simulink model "Energy_consumption_model_V3"  (R2022b)
settings: Solver=VariableStepAuto  StartTime=0.0  StopTime=110  RelTol=1e-3
undefined symbols (not defined in the file or in its folder): arr_db, arr_fg, arr_l, arr_lm, arr_mc1, arr_mc2, arr_mc3, arr_mc4, arr_mc5, arr_rg1, arr_rg2, arr_wc, EC_db, EC_fg, EC_l, EC_lm, EC_mc1, EC_mc2, EC_mc3, EC_mc4, EC_mc5, EC_rg1, EC_rg2, EC_wc, m, msg1, msg2, msg3, msg4, msg5, msgdb, msgfg, msgl, msglm, msgrg1, msgrg2, msgwc, n
(part 1 of 2)
settings Model: PacingRate=1000  Creator=Malar  LastModifiedBy=asogw
settings DataIOCC: InspectSignalLogs=on  LoggingToFile=on

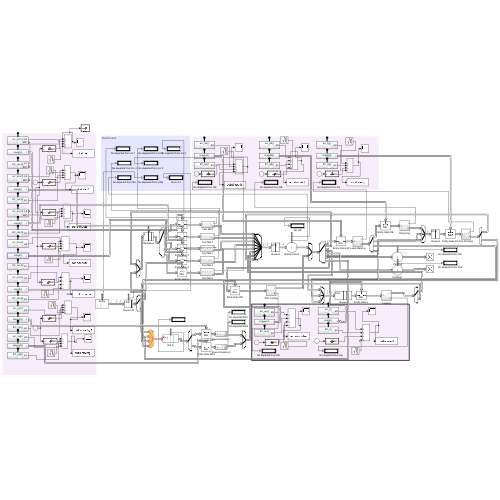
[thumbnail: Simulink's stored preview of the top-level diagram]
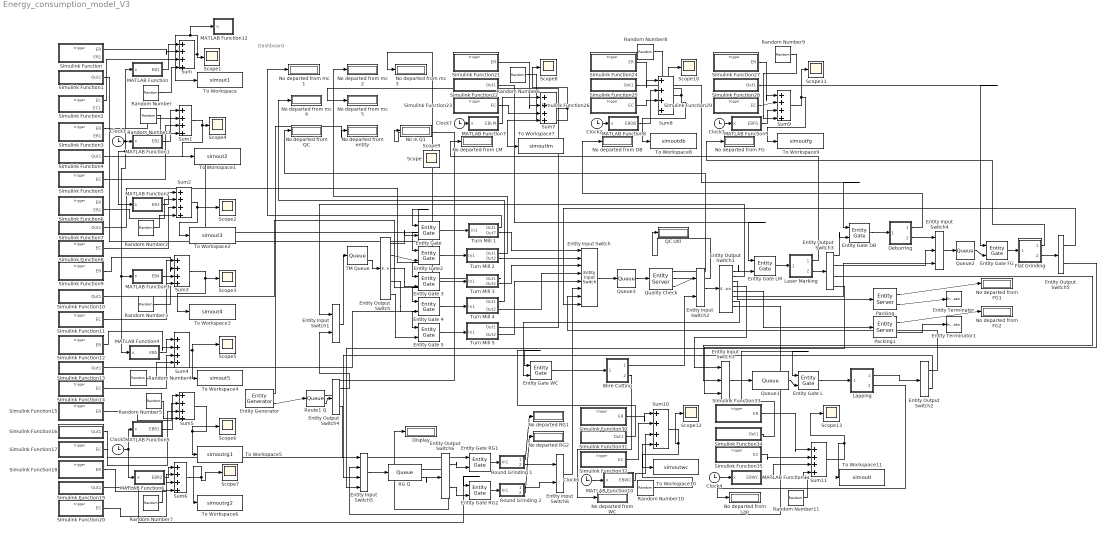
== system Energy_consumption_model_V3 ==
  note: Dashboard
  " Queue1" : Queue  InputPortMessageModes=m  OutputPortMessageModes=m  EntryAction=|
      | Ds= [2 0.2 ; 1 0.8];
      | 
      | rnum=rand();
      | for i=1:size(Ds,1)
      | if rnum<=sum(Ds(1:i,2))
      | entity.QualityCheck=Ds(i,1);
      | break
      | end
      | end
  " Queue2" : Queue  InputPortMessageModes=m  OutputPortMessageModes=m  EntryAction=|
      | Ds= [2 0.2 ; 1 0.8];
      | 
      | rnum=rand();
      | for i=1:size(Ds,1)
      | if rnum<=sum(Ds(1:i,2))
      | entity.QualityCheck=Ds(i,1);
      | break
      | end
      | end
  " Queue3" : Queue  InputPortMessageModes=m  OutputPortMessageModes=m  Capacity=50  EntryAction=|
      | %Ds= [2 0.2 ; 1 0.8];
      | 
      | %rnum=rand();
      | %for i=1:size(Ds,1)
      | %if rnum<=sum(Ds(1:i,2))
      | %entity.QualityCheck=Ds(i,1);
      | %break
      | %end
      | %end
  Clock{1..7} (7 alike) : Clock
  Deburring : Subsystem
  Display : Display
  Entity Input Switch : EntityInputSwitch  InputPortMessageModes=m,m,m,m,m,m,m,m  OutputPortMessageModes=m  NumberInputPorts=8
      settings: InputPortMap=u1,u2,u3,u4,u5,u6,u7,u8
  Entity Input Switch1 : EntityInputSwitch  InputPortMessageModes=m,m  OutputPortMessageModes=m
  Entity Input Switch2 : EntityInputSwitch  InputPortMessageModes=m,m  OutputPortMessageModes=m
  Entity Input Switch3 : EntityInputSwitch  InputPortMessageModes=m,m,m  OutputPortMessageModes=m  NumberInputPorts=3
      settings: InputPortMap=u1,u2,u3
  Entity Input Switch4 : EntityInputSwitch  InputPortMessageModes=m,m,m  OutputPortMessageModes=m  NumberInputPorts=3
      settings: InputPortMap=u1,u2,u3
  Entity Input Switch5 : EntityInputSwitch  InputPortMessageModes=m,m,m,m  OutputPortMessageModes=m  NumberInputPorts=4
      settings: InputPortMap=u1,u2,u3,u4
  Entity Input Switch6 : EntityInputSwitch  InputPortMessageModes=m,m  OutputPortMessageModes=m
  Entity Output Switch : EntityOutputSwitch  InputPortMessageModes=m  OutputPortMessageModes=m,m,m,m,m  NumberOutputPorts=5  SwitchAttributeName=Attribute1
      settings: OutputPortMap=o0,o1,o2,o3,o4
  Entity Output Switch1 : EntityOutputSwitch  InputPortMessageModes=m  OutputPortMessageModes=m,m,m,m,m,m,m,m  NumberOutputPorts=8  SwitchingCriterion=From attribute  SwitchAttributeName=Route
      settings: OutputPortMap=o0,o1,o2,o3,o4,o5,o6,o7
  Entity Output Switch2 : EntityOutputSwitch  InputPortMessageModes=m  OutputPortMessageModes=m,m  SwitchingCriterion=From attribute  SwitchAttributeName=Route
  Entity Output Switch3 : EntityOutputSwitch  InputPortMessageModes=m  OutputPortMessageModes=m,m,m,m  NumberOutputPorts=4  SwitchingCriterion=From attribute  SwitchAttributeName=Route
      settings: OutputPortMap=o0,o1,o2,o3
  Entity Output Switch4 : EntityOutputSwitch  InputPortMessageModes=m  OutputPortMessageModes=m,m  SwitchingCriterion=From attribute  SwitchAttributeName=Route
  Entity Output Switch5 : EntityOutputSwitch  InputPortMessageModes=m  OutputPortMessageModes=m,m  SwitchingCriterion=From attribute  SwitchAttributeName=Route
  Entity Output Switch6 : EntityOutputSwitch  InputPortMessageModes=m  OutputPortMessageModes=m,m  SwitchAttributeName=Route
  Entity Gate : EntityGate  InputPortMessageModes=m,m  OutputPortMessageModes=m  OperatingMode=Release gate  OpenGateAtSimulationStart=on
  Entity Gate 3 : EntityGate  InputPortMessageModes=m,m  OutputPortMessageModes=m  OperatingMode=Release gate  OpenGateAtSimulationStart=on
  Entity Gate 4 : EntityGate  InputPortMessageModes=m,m  OutputPortMessageModes=m  OperatingMode=Release gate  OpenGateAtSimulationStart=on
  Entity Gate 5 : EntityGate  InputPortMessageModes=m,m  OutputPortMessageModes=m  OperatingMode=Release gate  OpenGateAtSimulationStart=on
  Entity Gate DB : EntityGate  InputPortMessageModes=m,m  OutputPortMessageModes=m  OperatingMode=Release gate  OpenGateAtSimulationStart=on
  Entity Gate FG : EntityGate  InputPortMessageModes=m,m  OutputPortMessageModes=m  OperatingMode=Release gate  OpenGateAtSimulationStart=on
  Entity Gate L : EntityGate  InputPortMessageModes=m,m  OutputPortMessageModes=m  OperatingMode=Release gate  OpenGateAtSimulationStart=on
  Entity Gate LM : EntityGate  InputPortMessageModes=m,m  OutputPortMessageModes=m  OperatingMode=Release gate  OpenGateAtSimulationStart=on
  Entity Gate RG1 : EntityGate  InputPortMessageModes=m,m  OutputPortMessageModes=m  OperatingMode=Release gate  OpenGateAtSimulationStart=on
  Entity Gate RG2 : EntityGate  InputPortMessageModes=m,m  OutputPortMessageModes=m  OperatingMode=Release gate  OpenGateAtSimulationStart=on
  Entity Gate WC : EntityGate  InputPortMessageModes=m,m  OutputPortMessageModes=m  OperatingMode=Release gate  OpenGateAtSimulationStart=on
  Entity Gate2 : EntityGate  InputPortMessageModes=m,m  OutputPortMessageModes=m  OperatingMode=Release gate  OpenGateAtSimulationStart=on
  Entity Generator : EntityGenerator  OutputPortMessageModes=n,m  TimeSource=MATLAB action  IntergenerationTimeAction=|  GenerateAction=entitySys.priority=1000;  AttributeName=QualityCheck|Variant|Route|TMQC|Counter|ST|Time|PartCounter|Demand|Gate  AttributeInitialValue=0|1|1|0|0|0|1|0|0|0  NumberEntitiesDeparted=on  EntityType=Structured  EntityTypeName=Entity
      | %rng('shuffle');
      | dt = rand(1,1)*3;
      settings: OutputPortMap=o0,o3
  Entity Terminator : EntityTerminator  InputPortMessageModes=m
  Entity Terminator1 : EntityTerminator  InputPortMessageModes=m
  Flat Grinding : Subsystem
  Lapping : Subsystem
  Laser Marking : Subsystem
  MATLAB Function : MATLAB Function  TreatAsAtomicUnit=on
  MATLAB Function1 : MATLAB Function  TreatAsAtomicUnit=on
  MATLAB Function10 : MATLAB Function  TreatAsAtomicUnit=on
  MATLAB Function11 : MATLAB Function  TreatAsAtomicUnit=on
  MATLAB Function12 : MATLAB Function  TreatAsAtomicUnit=on
  MATLAB Function2 : MATLAB Function  TreatAsAtomicUnit=on
  MATLAB Function3 : MATLAB Function  TreatAsAtomicUnit=on
  MATLAB Function4 : MATLAB Function  TreatAsAtomicUnit=on
  MATLAB Function5 : MATLAB Function  TreatAsAtomicUnit=on
  MATLAB Function6 : MATLAB Function  TreatAsAtomicUnit=on
  MATLAB Function7 : MATLAB Function  TreatAsAtomicUnit=on
  MATLAB Function8 : MATLAB Function  TreatAsAtomicUnit=on
  MATLAB Function9 : MATLAB Function  TreatAsAtomicUnit=on
  No departed RG1 : Display
  No departed RG2 : Display
  No departed from DB : Display
  No departed from FG : Display
  No departed from FG1 : Display
  No departed from FG2 : Display
  No departed from LM : Display
  No departed from Lap : Display
  No departed from QC : Display
  No departed from WC : Display
  No departed from entity : Display
  No departed from mc {1..5} (5 alike) : Display
  No in Q1 : Display
  Packing : EntityServer  InputPortMessageModes=m  OutputPortMessageModes=n,m  Capacity=1  NumberEntitiesDeparted=on
      settings: OutputPortMap=o0,o9
  Packing1 : EntityServer  InputPortMessageModes=m  OutputPortMessageModes=n,m  Capacity=1  ServiceTimeValue=0  NumberEntitiesDeparted=on
      settings: OutputPortMap=o0,o9
  QC Util : Display
  Quality Check : EntityServer  InputPortMessageModes=m  OutputPortMessageModes=n,n,m  Capacity=1  ServiceTimeSource=MATLAB action  ServiceTimeAction=|  EntryAction=|  NumberEntitiesDeparted=on  Utilization=on
      ServiceTimeAction=|
      | coder.extrinsic("makedist")
      | pd = double(10)
      |  %rng('shuffle');
      | pd=random(makedist('Triangular','a',0.5,'b',1.9,'c',6),[1,1]);
      | dt = pd;
      EntryAction=|
      | r = rand(1,1)
      | if (entity.Variant == 8 & r < 0.95) %If variant = 8, then part rework happens 5% of the time 
      |     entity.Counter = entity.Counter + 1
      |     entity.QualityCheck = 2
      | elseif entity.Variant == 8
      |     entity.Counter = entity.Counter + 1
      |     entity.QualityCheck = 1
      | end
      | 
      | if (entity.Variant ~= 8 & r < 0.95) % If variant is not equal to 8, then two different QC are done (Passes both)
      |     entity.Counter = entity.Counter + 1 % The first QC is for Turning and Milling. 
      |     if entity.Counter == 1
      |         entity.TMQC = 2 %Pass TMQC
      |     elseif (entity.TMQC == 2 & entity.Counter == 2)
      |         entity.QualityCheck = 2 % Pass QC if coming for second time (This will be final inspection)
      |     end
      | elseif (entity.Variant ~= 8)% 5% of parts are sent to rework
      |     entity.Counter = entity.Counter + 1
      |     if entity.Counter == 1
      |         entity.TMQC = 1 %Fails TMQC
      |     elseif (entity.TMQC == 2 & entity.Counter == 2)
      |         entity.QualityCheck = 1 %Fails final QC
      |     end
      | end
      | 
      | 
      | %Part fails if the QualityCheck is 1 Pass if 2
      | if entity.Variant == 8
      |     if entity.QualityCheck == 1 
      |         entitySys.priority=1
      |         entity.Route = 8
      |     elseif entity.QualityCheck == 2
      |         entity.Route = 3
      |     end
      | elseif (entity.Variant == 9 & entity.TMQC == 2)
      |    if entity.Counter == 2
      |         entity.Route = 7  
      |    else
      |         entity.Route = 6
      |    end       
      | elseif entity.TMQC == 1 % Go to rework - back to TM
      |        entity.Route = 2
      | elseif entity.TMQC == 2 & entity.Variant == 7
      |         entity.Route = 5  
      | elseif entity.TMQC == 2 & entity.QualityCheck == 2 % Part pass QC - pack
      |         entity.Route = 3
      | else % TMQC pass Go to laser marking
      |         entity.Route = 1
      | end
      settings: OutputPortMap=o0,o5,o9
  RG Q : Queue  InputPortMessageModes=m  OutputPortMessageModes=n,m  QueueType=Priority  PrioritySource=entitySys.priority  NumberEntitiesInBlock=on
      settings: OutputPortMap=o1,o5
  Random Number : RandomNumber  Variance=30  Seed=11  SampleTime=1
  Random Number1 : RandomNumber  Variance=30  Seed=22  SampleTime=1
  Random Number10 : RandomNumber  Variance=30  Seed=88  SampleTime=1
  Random Number11 : RandomNumber  Variance=30  Seed=99  SampleTime=1
  Random Number2 : RandomNumber  Variance=30  Seed=33  SampleTime=1
  Random Number3 : RandomNumber  Variance=30  Seed=44  SampleTime=1
  Random Number4 : RandomNumber  Variance=30  Seed=55  SampleTime=1
  Random Number5 : RandomNumber  Variance=30  Seed=66  SampleTime=1
  Random Number6 : RandomNumber  Variance=30  Seed=22  SampleTime=1
  Random Number7 : RandomNumber  Variance=30  Seed=77  SampleTime=1
  Random Number8 : RandomNumber  Variance=30  Seed=33  SampleTime=1
  Random Number9 : RandomNumber  Variance=30  Seed=1  SampleTime=1
  Round Grinding 1 : Subsystem
  Round Grinding 2 : Subsystem
  Route1 Q : Queue  InputPortMessageModes=m  OutputPortMessageModes=n,m  EntryAction=|  NumberEntitiesInBlock=on
      | %rng('shuffle');
      | t = rand(1,1);
      | if t <= 0.41
      |     entity.Variant =1;
      | elseif t <= 0.45
      |     entity.Variant = 2;
      | elseif t <= 0.567
      |     entity.Variant = 3;
      | elseif t <= 0.645
      |     entity.Variant = 4;
      | elseif t <= 0.685
      |     entity.Variant = 5;
      | elseif t <= 0.841
      |     entity.Variant = 6;
      | elseif t <= 0.90
      |     entity.Variant = 7;
      | elseif t <= 0.92
      |     entity.Variant = 8;
      |      entity.Route = 2;
      | elseif t <= 0.96
      |     entity.Variant = 9;
      | else
      |     entity.Variant = 10;
      | end
      settings: OutputPortMap=o1,o5
  Scope{,1..13} (14 alike) : Scope
  Simulink Function : Subsystem  TreatAsAtomicUnit=on
  Simulink Function1 : Subsystem  TreatAsAtomicUnit=on
  Simulink Function10 : Subsystem  TreatAsAtomicUnit=on
  Simulink Function11 : Subsystem  TreatAsAtomicUnit=on
  Simulink Function12 : Subsystem  TreatAsAtomicUnit=on
  Simulink Function13 : Subsystem  TreatAsAtomicUnit=on
  Simulink Function14 : Subsystem  TreatAsAtomicUnit=on
  Simulink Function15 : Subsystem  TreatAsAtomicUnit=on
  Simulink Function16 : Subsystem  TreatAsAtomicUnit=on
  Simulink Function17 : Subsystem  TreatAsAtomicUnit=on
  Simulink Function18 : Subsystem  TreatAsAtomicUnit=on
  Simulink Function19 : Subsystem  TreatAsAtomicUnit=on
  Simulink Function2 : Subsystem  TreatAsAtomicUnit=on
  Simulink Function20 : Subsystem  TreatAsAtomicUnit=on
  Simulink Function21 : Subsystem  TreatAsAtomicUnit=on
  Simulink Function22 : Subsystem  TreatAsAtomicUnit=on
  Simulink Function23 : Subsystem  TreatAsAtomicUnit=on
  Simulink Function24 : Subsystem  TreatAsAtomicUnit=on
  Simulink Function25 : Subsystem  TreatAsAtomicUnit=on
  Simulink Function26 : Subsystem  TreatAsAtomicUnit=on
  Simulink Function27 : Subsystem  TreatAsAtomicUnit=on
  Simulink Function28 : Subsystem  TreatAsAtomicUnit=on
  Simulink Function29 : Subsystem  TreatAsAtomicUnit=on
  Simulink Function3 : Subsystem  TreatAsAtomicUnit=on
  Simulink Function30 : Subsystem  TreatAsAtomicUnit=on
  Simulink Function31 : Subsystem  TreatAsAtomicUnit=on
  Simulink Function32 : Subsystem  TreatAsAtomicUnit=on
  Simulink Function33 : Subsystem  TreatAsAtomicUnit=on
  Simulink Function34 : Subsystem  TreatAsAtomicUnit=on
  Simulink Function35 : Subsystem  TreatAsAtomicUnit=on
  Simulink Function4 : Subsystem  TreatAsAtomicUnit=on
  Simulink Function5 : Subsystem  TreatAsAtomicUnit=on
  Simulink Function6 : Subsystem  TreatAsAtomicUnit=on
  Simulink Function7 : Subsystem  TreatAsAtomicUnit=on
  Simulink Function8 : Subsystem  TreatAsAtomicUnit=on
  Simulink Function9 : Subsystem  TreatAsAtomicUnit=on
  Sum{,1..11} (12 alike) : Sum  Inputs=|++++
  TM Queue : Queue  InputPortMessageModes=m  OutputPortMessageModes=n,m  Capacity=50  QueueType=Priority  PrioritySource=entitySys.priority  NumberEntitiesInBlock=on
      settings: OutputPortMap=o1,o5
  To Workspace : ToWorkspace  VariableName=simout1  SampleTime=-1
  To Workspace1 : ToWorkspace  VariableName=simout2  SampleTime=-1
  To Workspace10 : ToWorkspace  VariableName=simoutwc  SampleTime=-1
  To Workspace11 : ToWorkspace  VariableName=simoutl  SampleTime=-1
  To Workspace2 : ToWorkspace  VariableName=simout3  SampleTime=-1
  To Workspace3 : ToWorkspace  VariableName=simout4  SampleTime=-1
  To Workspace4 : ToWorkspace  VariableName=simout5  SampleTime=-1
  To Workspace5 : ToWorkspace  VariableName=simoutrg1  SampleTime=-1
  To Workspace6 : ToWorkspace  VariableName=simoutrg2  SampleTime=-1
  To Workspace7 : ToWorkspace  VariableName=simoutlm  SampleTime=-1
  To Workspace8 : ToWorkspace  VariableName=simoutdb  SampleTime=-1
  To Workspace9 : ToWorkspace  VariableName=simoutfg  SampleTime=-1
  Turn Mill 1 : Subsystem
  Turn Mill 2 : Subsystem
  Turn Mill 3 : Subsystem
  Turn Mill 4 : Subsystem
  Turn Mill 5 : Subsystem
  Wire Cutting : Subsystem
  wires:
  Entity Input Switch/1 -> " Queue3"/1
  Entity Output Switch1/3 -> Packing/1
  " Queue3"/1 -> Quality Check/1
  Entity Input Switch3/1 -> " Queue1"/1
  Entity Output Switch1/4 -> Entity Input Switch3/1
  Entity Output Switch3/3 -> Entity Input Switch3/2
  Entity Input Switch4/1 -> " Queue2"/1
  Entity Output Switch3/2 -> Entity Input Switch4/2
  Route1 Q/2 -> Entity Output Switch4/1
  RG Q/1 -> Display/1
  Entity Input Switch5/1 -> RG Q/1
  Entity Output Switch4/2 -> Entity Input Switch5/1
  Entity Output Switch1/8 -> Entity Input Switch5/2
  Packing/2 -> Entity Terminator/1
  Entity Output Switch2/1 -> Entity Input Switch/7
  TM Queue/2 -> Entity Output Switch/1
  Entity Input Switch1/1 -> TM Queue/1
  Entity Output Switch2/2 -> Entity Input Switch5/3
  Entity Output Switch4/1 -> Entity Input Switch1/2
  Entity Output Switch1/2 -> Entity Input Switch1/1
  Entity Output Switch5/1 -> Entity Input Switch/8
  Entity Output Switch5/2 -> Entity Input Switch3/3
  Entity Output Switch1/6 -> Entity Input Switch4/3
  Entity Output Switch1/7 -> Entity Gate WC/2
  Entity Input Switch2/1 -> Entity Output Switch1/1
  Quality Check/3 -> Entity Input Switch2/1
  Entity Output Switch3/4 -> Entity Input Switch5/4
  RG Q/2 -> Entity Output Switch6/1
  Entity Input Switch6/1 -> Entity Input Switch/6
  Quality Check/2 -> QC Util/1
  Quality Check/1 -> No departed from QC/1
  Entity Output Switch/1 -> Entity Gate/2
  MATLAB Function/1(EB1) -> Sum/1
  Sum/1 -> Scope1/1, MATLAB Function12/1(u), To Workspace/1
  Simulink Function/1(ER) -> Sum/2
  Simulink Function1/1(Out1) -> Entity Gate/1
  Simulink Function2/1(EC) -> Sum/3
  Entity Gate/1 -> Turn Mill 1/1(In1)
  Turn Mill 1/1(Out1) -> No departed from mc 1/1
  Turn Mill 1/2(Out7) -> Entity Input Switch/1
  Clock1/1 -> MATLAB Function4/1(x), MATLAB Function3/1(x), MATLAB Function2/1(x), MATLAB Function/1(x), MATLAB Function1/1(x)
  Turn Mill 2/1(Out1) -> No departed from mc 2/1
  Turn Mill 2/2(Out2) -> Entity Input Switch/2
  Simulink Function4/1(Out1) -> Entity Gate2/1
  Entity Output Switch/2 -> Entity Gate2/2
  Entity Gate2/1 -> Turn Mill 2/1(In1)
  Simulink Function3/1(ER) -> Sum1/2
  MATLAB Function1/1(EB2) -> Sum1/1
  Simulink Function5/1(EC) -> Sum1/3
  Sum1/1 -> To Workspace1/1, Scope4/1
  Entity Output Switch/3 -> Entity Gate 3/2
  Simulink Function7/1(Out1) -> Entity Gate 3/1
  Entity Gate 3/1 -> Turn Mill 3/1(In1)
  Turn Mill 3/1(Out1) -> No departed from mc 3/1
  Turn Mill 3/2(Out2) -> Entity Input Switch/3
  MATLAB Function2/1(EB3) -> Sum2/1
  Simulink Function6/2(ER1) -> Sum2/2
  Simulink Function8/1(EC) -> Sum2/3
  Sum2/1 -> Scope2/1, To Workspace2/1
  Entity Output Switch/4 -> Entity Gate 4/2
  Simulink Function10/1(Out1) -> Entity Gate 4/1
  Entity Gate 4/1 -> Turn Mill 4/1(In1)
  Turn Mill 4/1(Out1) -> No departed from mc 4/1
  Turn Mill 4/2(Out2) -> Entity Input Switch/4
  MATLAB Function3/1(EB4) -> Sum3/1
  Simulink Function9/1(ER) -> Sum3/2
  Simulink Function11/1(EC) -> Sum3/3
  Sum3/1 -> To Workspace3/1, Scope3/1
  Entity Output Switch/5 -> Entity Gate 5/2
  MATLAB Function4/1(EB5) -> Sum4/1
  Sum4/1 -> To Workspace4/1, Scope5/1
  Entity Gate 5/1 -> Turn Mill 5/1(In1)
  Turn Mill 5/1(Out1) -> No departed from mc 5/1
  Turn Mill 5/2(Out2) -> Entity Input Switch/5
  Simulink Function13/1(Out1) -> Entity Gate 5/1
  Simulink Function12/1(ER) -> Sum4/2
  Simulink Function14/1(EC) -> Sum4/3
  Entity Output Switch6/1 -> Entity Gate RG1/2
  Entity Gate RG1/1 -> Round Grinding 1/1(In1)
  Round Grinding 1/1(Out1) -> No departed RG1/1
  Round Grinding 1/2(Out2) -> Entity Input Switch6/1
  Clock5/1 -> MATLAB Function6/1(x), MATLAB Function5/1(x)
  MATLAB Function5/1(EBR1) -> Sum5/1
  Sum5/1 -> To Workspace5/1, Scope6/1
  Simulink Function16/1(Out1) -> Entity Gate RG1/1
  Simulink Function15/1(ER) -> Sum5/2
  Simulink Function17/1(EC) -> Sum5/3
  MATLAB Function6/1(EBR2) -> Sum6/1
  Sum6/1 -> Scope7/1, To Workspace6/1
  Simulink Function18/1(ER) -> Sum6/2
  Simulink Function19/1(Out1) -> Entity Gate RG2/1
  Entity Output Switch6/2 -> Entity Gate RG2/2
  Entity Gate RG2/1 -> Round Grinding 2/1(In1)
  Round Grinding 2/1(Out1) -> Entity Input Switch6/2
  Simulink Function20/1(EC) -> Sum6/3
  Round Grinding 2/2(Out2) -> No departed RG2/1
  Entity Output Switch1/1 -> Entity Gate LM/2
  Simulink Function22/1(Out1) -> Entity Gate LM/1
  Entity Gate LM/1 -> Laser Marking/1(In1)
  Laser Marking/2(Out2) -> Entity Output Switch3/1
  Laser Marking/1(Out1) -> No departed from LM/1
  Clock7/1 -> MATLAB Function7/1(x)
  MATLAB Function7/1(EBLM) -> Sum7/1
  Simulink Function21/1(ER) -> Sum7/2
  Simulink Function23/1(EC) -> Sum7/3
  Sum7/1 -> Scope8/1, To Workspace7/1
  Clock2/1 -> MATLAB Function8/1(x)
  Simulink Function24/1(ER) -> Sum8/1
  MATLAB Function8/1(EBDB) -> Sum8/2
  Simulink Function26/1(EC) -> Sum8/3
  Simulink Function25/1(Out1) -> Entity Gate DB/1
  Entity Output Switch3/1 -> Entity Gate DB/2
  Entity Gate DB/1 -> Deburring/1(In1)
  Deburring/1(Out1) -> No departed from DB/1
  Deburring/2(Out2) -> Entity Input Switch4/1
  Sum8/1 -> To Workspace8/1, Scope10/1
  " Queue2"/1 -> Entity Gate FG/2
  Clock3/1 -> MATLAB Function9/1(x)
  Simulink Function27/1(ER) -> Sum9/1
  Simulink Function29/1(EC) -> Sum9/2
  MATLAB Function9/1(EBFG) -> Sum9/3
  Sum9/1 -> Scope11/1, To Workspace9/1
  Entity Gate FG/1 -> Flat Grinding/1(In1)
  Flat Grinding/1(Out1) -> No departed from FG/1
  Flat Grinding/2(Out2) -> Entity Output Switch5/1
  Simulink Function28/1(Out1) -> Entity Gate FG/1
  Clock6/1 -> MATLAB Function10/1(x)
  Simulink Function30/1(ER) -> Sum10/1
  Simulink Function32/1(EC) -> Sum10/2
  MATLAB Function10/1(EBWC) -> Sum10/3
  Simulink Function31/1(Out1) -> Entity Gate WC/1
  Sum10/1 -> Scope12/1, To Workspace10/1
  Entity Gate WC/1 -> Wire Cutting/1(In1)
  Wire Cutting/1(Out1) -> Entity Input Switch2/2
  Wire Cutting/2(Out2) -> No departed from WC/1
  Clock4/1 -> MATLAB Function11/1(x)
  Sum11/1 -> Scope13/1, To Workspace11/1
  MATLAB Function11/1(EBWC) -> Sum11/3
  Simulink Function35/1(EC) -> Sum11/2
  Simulink Function33/1(ER) -> Sum11/1
  " Queue1"/1 -> Entity Gate L/2
  Simulink Function34/1(Out1) -> Entity Gate L/1
  Entity Gate L/1 -> Lapping/1(In1)
  Lapping/1(Out1) -> Entity Output Switch2/1
  Lapping/2(Out2) -> No departed from Lap/1
  Random Number/1 -> Sum/4
  Random Number1/1 -> Sum1/4
  Random Number2/1 -> Sum2/4
  Random Number3/1 -> Sum3/4
  Random Number4/1 -> Sum4/4
  Random Number5/1 -> Sum5/4
  Random Number6/1 -> Sum7/4
  Random Number7/1 -> Sum6/4
  Random Number8/1 -> Sum8/4
  Random Number9/1 -> Sum9/4
  Random Number10/1 -> Sum10/4
  Random Number11/1 -> Sum11/4
  Entity Generator/2 -> Route1 Q/1
  Packing/1 -> No departed from FG1/1
  Packing1/2 -> Entity Terminator1/1
  Entity Output Switch1/5 -> Packing1/1
  Packing1/1 -> No departed from FG2/1
  Entity Generator/1 -> No departed from entity/1
  Route1 Q/1 -> No in Q1/1

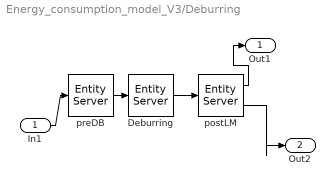
== system Energy_consumption_model_V3/Deburring ==
  In1 : Inport
  Deburring : EntityServer  InputPortMessageModes=m  OutputPortMessageModes=m  Capacity=1  ServiceTimeSource=MATLAB action  ServiceTimeAction=|  EntryAction=EC_db()  ServiceCompleteAction=EC_db()
      | coder.extrinsic("makedist")
      | pd = double(10)
      | pd=random(makedist('Triangular','a',0.75,'b',2.15,'c',2.75),[1,1])
      | dt = pd
  postLM : EntityServer  InputPortMessageModes=m  OutputPortMessageModes=n,m  Capacity=1  ServiceTimeSource=MATLAB action  ServiceTimeAction=dt = 0.25;  ServiceCompleteAction=arr_db()  ExitAction=msgdb()  NumberEntitiesDeparted=on
      settings: OutputPortMap=o0,o9
  preDB : EntityServer  InputPortMessageModes=m  OutputPortMessageModes=m  Capacity=1  ServiceTimeSource=MATLAB action  ServiceTimeAction=dt = 0.25;  EntryAction=arr_db()
  Out1 : Outport
  Out2 : Outport  Port=2
  wires:
  preDB/1 -> Deburring/1
  postLM/1 -> Out1/1
  postLM/2 -> Out2/1
  In1/1 -> preDB/1
  Deburring/1 -> postLM/1

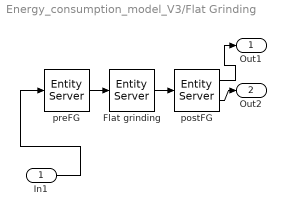
== system Energy_consumption_model_V3/Flat Grinding ==
  In1 : Inport
  Flat grinding : EntityServer  InputPortMessageModes=m  OutputPortMessageModes=m  Capacity=1  ServiceTimeSource=MATLAB action  ServiceTimeAction=|  EntryAction=|  ServiceCompleteAction=EC_fg()
      ServiceTimeAction=|
      | coder.extrinsic("makedist")
      | pd = double(10)
      | pd=random(makedist('Triangular','a',0.5,'b',1.5,'c',5),[1,1])
      | dt = pd
      EntryAction=|
      | if (entity.Variant == 2 | entity.Variant == 4)
      |     entity.Route = 1
      | elseif (entity.Variant == 3 | entity.Variant == 5 | entity.Variant == 9 )
      |     entity.Route = 2
      | end
      | 
      | EC_fg()
  postFG : EntityServer  InputPortMessageModes=m  OutputPortMessageModes=n,m  Capacity=1  ServiceTimeSource=MATLAB action  ServiceTimeAction=dt = 0.10;  ServiceCompleteAction=arr_fg()  ExitAction=msgfg()  NumberEntitiesDeparted=on
      settings: OutputPortMap=o0,o9
  preFG : EntityServer  InputPortMessageModes=m  OutputPortMessageModes=m  Capacity=1  ServiceTimeSource=MATLAB action  ServiceTimeAction=dt = 0.10;  EntryAction=arr_fg()
  Out1 : Outport
  Out2 : Outport  Port=2
  wires:
  preFG/1 -> Flat grinding/1
  Flat grinding/1 -> postFG/1
  postFG/1 -> Out1/1
  postFG/2 -> Out2/1
  In1/1 -> preFG/1

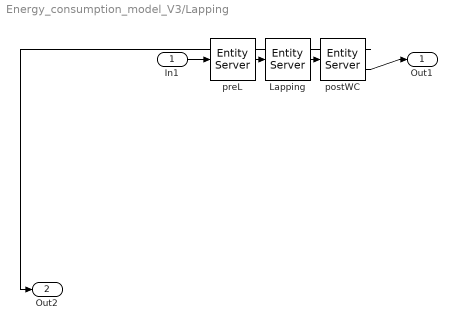
== system Energy_consumption_model_V3/Lapping ==
  In1 : Inport
  Lapping : EntityServer  InputPortMessageModes=m  OutputPortMessageModes=m  Capacity=1  ServiceTimeSource=MATLAB action  ServiceTimeAction=|  EntryAction=|  ServiceCompleteAction=EC_l()
      ServiceTimeAction=|
      | coder.extrinsic("makedist")
      | pd = double(10)
      | pd=random(makedist('Triangular','a',0.5,'b',1.76,'c',3),[1,1])
      | dt = pd
      EntryAction=|
      | entitySys.priority=50
      | if (entity.Variant == 1 | entity.Variant == 3 | entity.Variant == 5)
      |     entity.Route = 2
      | elseif (entity.Variant == 6 | entity.Variant == 9)
      |     entity.Route = 1
      | end
      | EC_l()
  postWC : EntityServer  InputPortMessageModes=m  OutputPortMessageModes=n,m  Capacity=1  ServiceTimeSource=MATLAB action  ServiceTimeAction=dt = 0.10;  ServiceCompleteAction=arr_l()  ExitAction=msgl()  NumberEntitiesDeparted=on
      settings: OutputPortMap=o0,o9
  preL : EntityServer  InputPortMessageModes=m  OutputPortMessageModes=m  Capacity=1  ServiceTimeSource=MATLAB action  ServiceTimeAction=dt = 0.10;  EntryAction=arr_l()
  Out1 : Outport
  Out2 : Outport  Port=2
  wires:
  postWC/2 -> Out1/1
  preL/1 -> Lapping/1
  Lapping/1 -> postWC/1
  In1/1 -> preL/1
  postWC/1 -> Out2/1

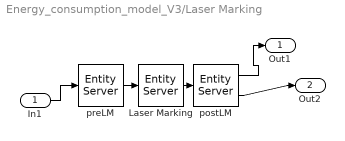
== system Energy_consumption_model_V3/Laser Marking ==
  In1 : Inport
  Laser Marking : EntityServer  InputPortMessageModes=m  OutputPortMessageModes=m  Capacity=1  ServiceTimeSource=MATLAB action  ServiceTimeAction=|  EntryAction=|  ServiceCompleteAction=EC_lm()
      ServiceTimeAction=|
      | coder.extrinsic("makedist")
      | pd = double(10)
      | pd=random(makedist('Triangular','a',0.16,'b',0.88,'c',3),[1,1])
      | dt = pd
      EntryAction=|
      | if (entity.Variant == 1 | entity.Variant == 6)
      |     entity.Route = 3
      | elseif (entity.Variant == 2 | entity.Variant == 4)
      |     entity.Route = 2
      | elseif entity.Variant == 5
      |     entity.Route = 1
      | elseif entity.Variant == 10
      |     entity.Route = 4
      | end
      | 
      | EC_lm()
  postLM : EntityServer  InputPortMessageModes=m  OutputPortMessageModes=n,m  Capacity=1  ServiceTimeSource=MATLAB action  ServiceTimeAction=dt = 0.25;  ServiceCompleteAction=arr_lm()  ExitAction=msglm()  NumberEntitiesDeparted=on
      settings: OutputPortMap=o0,o9
  preLM : EntityServer  InputPortMessageModes=m  OutputPortMessageModes=m  Capacity=1  ServiceTimeSource=MATLAB action  ServiceTimeAction=dt = 0.10;  EntryAction=arr_lm()
  Out1 : Outport
  Out2 : Outport  Port=2
  wires:
  Laser Marking/1 -> postLM/1
  postLM/2 -> Out2/1
  postLM/1 -> Out1/1
  preLM/1 -> Laser Marking/1
  In1/1 -> preLM/1

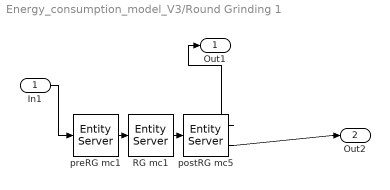
== system Energy_consumption_model_V3/Round Grinding 1 ==
  In1 : Inport
  RG mc1 : EntityServer  InputPortMessageModes=m  OutputPortMessageModes=m  Capacity=1  ServiceTimeSource=MATLAB action  ServiceTimeAttributeName=ST  ServiceTimeAction=|  EntryAction=EC_rg1()  ServiceCompleteAction=EC_rg1()
      | coder.extrinsic("makedist")
      | pd = double(10);
      |  %rng('shuffle');
      | pd=random(makedist('Triangular','a',0.25,'b',3.8,'c',4.75),[1,1]);
      | dt = pd;
  postRG mc5 : EntityServer  InputPortMessageModes=m  OutputPortMessageModes=n,m  Capacity=1  ServiceTimeSource=MATLAB action  ServiceTimeAction=dt = 0.25;  ServiceCompleteAction=arr_rg1()  ExitAction=msgrg1()  NumberEntitiesDeparted=on
      settings: OutputPortMap=o0,o9
  preRG mc1 : EntityServer  InputPortMessageModes=m  OutputPortMessageModes=m  Capacity=1  ServiceTimeSource=MATLAB action  ServiceTimeAction=dt = 0.25;  EntryAction=arr_rg1()
  Out1 : Outport
  Out2 : Outport  Port=2
  wires:
  preRG mc1/1 -> RG mc1/1
  RG mc1/1 -> postRG mc5/1
  In1/1 -> preRG mc1/1
  postRG mc5/1 -> Out1/1
  postRG mc5/2 -> Out2/1

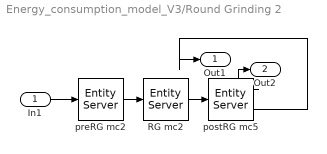
== system Energy_consumption_model_V3/Round Grinding 2 ==
  In1 : Inport
  RG mc2 : EntityServer  InputPortMessageModes=m  OutputPortMessageModes=m  Capacity=1  ServiceTimeSource=MATLAB action  ServiceTimeAction=|  EntryAction=EC_rg2()  ServiceCompleteAction=EC_rg2()
      | coder.extrinsic("makedist")
      | pd = double(10);
      |  %rng('shuffle');
      | pd=random(makedist('Triangular','a',1,'b',3.88,'c',4.75),[1,1]);
      | dt = pd;
  postRG mc5 : EntityServer  InputPortMessageModes=m  OutputPortMessageModes=n,m  Capacity=1  ServiceTimeSource=MATLAB action  ServiceTimeAction=dt = 0.25;  ServiceCompleteAction=arr_rg2()  ExitAction=msgrg2()  NumberEntitiesDeparted=on
      settings: OutputPortMap=o0,o9
  preRG mc2 : EntityServer  InputPortMessageModes=m  OutputPortMessageModes=m  Capacity=1  ServiceTimeSource=MATLAB action  ServiceTimeAction=dt = 0.25;  EntryAction=arr_rg2()
  Out1 : Outport
  Out2 : Outport  Port=2
  wires:
  preRG mc2/1 -> RG mc2/1
  In1/1 -> preRG mc2/1
  postRG mc5/1 -> Out2/1
  RG mc2/1 -> postRG mc5/1
  postRG mc5/2 -> Out1/1

== system Energy_consumption_model_V3/Simulink Function ==
  arr_mc1 : TriggerPort  TriggerType=function-call  IsSimulinkFunction=on  FunctionName=arr_mc1  FunctionVisibility=scoped  VariantControl=(inherit)
  Digital Clock : DigitalClock  SampleTime=-1
  MATLAB Function : MATLAB Function  TreatAsAtomicUnit=on
  ER : Outport
  ER1 : Outport  Port=2
  wires:
  Digital Clock/1 -> MATLAB Function/1(ct_ertm1)
  MATLAB Function/1(ERTM1) -> ER1/1, ER/1

== system Energy_consumption_model_V3/Simulink Function1 ==
  msg1 : TriggerPort  TriggerType=function-call  IsSimulinkFunction=on  FunctionName=msg1  FunctionVisibility=scoped  VariantControl=(inherit)
  Constant : Constant
  Send : Send  OutputPortMessageModes=m
  Out1 : Outport
  wires:
  Constant/1 -> Send/1
  Send/1 -> Out1/1

== system Energy_consumption_model_V3/Simulink Function10 ==
  msg4 : TriggerPort  TriggerType=function-call  IsSimulinkFunction=on  FunctionName=msg4  FunctionVisibility=scoped  VariantControl=(inherit)
  Constant : Constant
  Send : Send  OutputPortMessageModes=m
  Out1 : Outport
  wires:
  Constant/1 -> Send/1
  Send/1 -> Out1/1

== system Energy_consumption_model_V3/Simulink Function11 ==
  EC_mc4 : TriggerPort  TriggerType=function-call  IsSimulinkFunction=on  FunctionName=EC_mc4  FunctionVisibility=scoped  VariantControl=(inherit)
  Digital Clock : DigitalClock  SampleTime=-1
  MATLAB Function : MATLAB Function  TreatAsAtomicUnit=on
  EC : Outport
  wires:
  Digital Clock/1 -> MATLAB Function/1(ct_ectm4)
  MATLAB Function/1(ECTM4) -> EC/1

== system Energy_consumption_model_V3/Simulink Function12 ==
  arr_mc5 : TriggerPort  TriggerType=function-call  IsSimulinkFunction=on  FunctionName=arr_mc5  FunctionVisibility=scoped  VariantControl=(inherit)
  Digital Clock : DigitalClock  SampleTime=-1
  MATLAB Function : MATLAB Function  TreatAsAtomicUnit=on
  ER : Outport
  wires:
  Digital Clock/1 -> MATLAB Function/1(ct_ertm5)
  MATLAB Function/1(ERTM5) -> ER/1

== system Energy_consumption_model_V3/Simulink Function13 ==
  msg5 : TriggerPort  TriggerType=function-call  IsSimulinkFunction=on  FunctionName=msg5  FunctionVisibility=scoped  VariantControl=(inherit)
  Constant : Constant
  Send : Send  OutputPortMessageModes=m
  Out1 : Outport
  wires:
  Constant/1 -> Send/1
  Send/1 -> Out1/1

== system Energy_consumption_model_V3/Simulink Function14 ==
  EC_mc5 : TriggerPort  TriggerType=function-call  IsSimulinkFunction=on  FunctionName=EC_mc5  FunctionVisibility=scoped  VariantControl=(inherit)
  Digital Clock : DigitalClock  SampleTime=-1
  MATLAB Function : MATLAB Function  TreatAsAtomicUnit=on
  EC : Outport
  wires:
  Digital Clock/1 -> MATLAB Function/1(ct_ectm5)
  MATLAB Function/1(ECTM5) -> EC/1

== system Energy_consumption_model_V3/Simulink Function15 ==
  arr_rg1 : TriggerPort  TriggerType=function-call  IsSimulinkFunction=on  FunctionName=arr_rg1  FunctionVisibility=scoped  VariantControl=(inherit)
  Digital Clock : DigitalClock  SampleTime=-1
  MATLAB Function : MATLAB Function  TreatAsAtomicUnit=on
  ER : Outport
  wires:
  Digital Clock/1 -> MATLAB Function/1(ct_errg1)
  MATLAB Function/1(ERRG1) -> ER/1

== system Energy_consumption_model_V3/Simulink Function16 ==
  msgrg1 : TriggerPort  TriggerType=function-call  IsSimulinkFunction=on  FunctionName=msgrg1  FunctionVisibility=scoped  VariantControl=(inherit)
  Constant : Constant
  Send : Send  OutputPortMessageModes=m
  Out1 : Outport
  wires:
  Constant/1 -> Send/1
  Send/1 -> Out1/1

== system Energy_consumption_model_V3/Simulink Function17 ==
  EC_rg1 : TriggerPort  TriggerType=function-call  IsSimulinkFunction=on  FunctionName=EC_rg1  FunctionVisibility=scoped  VariantControl=(inherit)
  Digital Clock : DigitalClock  SampleTime=-1
  MATLAB Function : MATLAB Function  TreatAsAtomicUnit=on
  EC : Outport
  wires:
  Digital Clock/1 -> MATLAB Function/1(ct_ecrg1)
  MATLAB Function/1(ECRG1) -> EC/1

== system Energy_consumption_model_V3/Simulink Function18 ==
  arr_rg2 : TriggerPort  TriggerType=function-call  IsSimulinkFunction=on  FunctionName=arr_rg2  FunctionVisibility=scoped  VariantControl=(inherit)
  Digital Clock : DigitalClock  SampleTime=-1
  MATLAB Function : MATLAB Function  TreatAsAtomicUnit=on
  ER : Outport
  wires:
  Digital Clock/1 -> MATLAB Function/1(ct_errg2)
  MATLAB Function/1(ERRG2) -> ER/1

== system Energy_consumption_model_V3/Simulink Function19 ==
  msgrg2 : TriggerPort  TriggerType=function-call  IsSimulinkFunction=on  FunctionName=msgrg2  FunctionVisibility=scoped  VariantControl=(inherit)
  Constant : Constant
  Send : Send  OutputPortMessageModes=m
  Out1 : Outport
  wires:
  Constant/1 -> Send/1
  Send/1 -> Out1/1

== system Energy_consumption_model_V3/Simulink Function2 ==
  EC_mc1 : TriggerPort  TriggerType=function-call  IsSimulinkFunction=on  FunctionName=EC_mc1  FunctionVisibility=scoped  VariantControl=(inherit)
  Digital Clock : DigitalClock  SampleTime=-1
  MATLAB Function : MATLAB Function  TreatAsAtomicUnit=on
  EC : Outport
  EC1 : Outport  Port=2
  wires:
  Digital Clock/1 -> MATLAB Function/1(ct_ectm1)
  MATLAB Function/1(ECTM1) -> EC1/1, EC/1

== system Energy_consumption_model_V3/Simulink Function20 ==
  EC_rg2 : TriggerPort  TriggerType=function-call  IsSimulinkFunction=on  FunctionName=EC_rg2  FunctionVisibility=scoped  VariantControl=(inherit)
  Digital Clock : DigitalClock  SampleTime=-1
  MATLAB Function : MATLAB Function  TreatAsAtomicUnit=on
  EC : Outport
  wires:
  Digital Clock/1 -> MATLAB Function/1(ct_ecrg2)
  MATLAB Function/1(ECRG2) -> EC/1

== system Energy_consumption_model_V3/Simulink Function21 ==
  arr_lm : TriggerPort  TriggerType=function-call  IsSimulinkFunction=on  FunctionName=arr_lm  FunctionVisibility=scoped  VariantControl=(inherit)
  Digital Clock : DigitalClock  SampleTime=-1
  MATLAB Function : MATLAB Function  TreatAsAtomicUnit=on
  ER : Outport
  wires:
  Digital Clock/1 -> MATLAB Function/1(ct_erlm)
  MATLAB Function/1(ERLM) -> ER/1

== system Energy_consumption_model_V3/Simulink Function22 ==
  msglm : TriggerPort  TriggerType=function-call  IsSimulinkFunction=on  FunctionName=msglm  FunctionVisibility=scoped  VariantControl=(inherit)
  Constant : Constant
  Send : Send  OutputPortMessageModes=m
  Out1 : Outport
  wires:
  Constant/1 -> Send/1
  Send/1 -> Out1/1

== system Energy_consumption_model_V3/Simulink Function23 ==
  EC_lm : TriggerPort  TriggerType=function-call  IsSimulinkFunction=on  FunctionName=EC_lm  FunctionVisibility=scoped  VariantControl=(inherit)
  Digital Clock : DigitalClock  SampleTime=-1
  MATLAB Function : MATLAB Function  TreatAsAtomicUnit=on
  EC : Outport
  wires:
  Digital Clock/1 -> MATLAB Function/1(ct_eclm)
  MATLAB Function/1(ECLM) -> EC/1

== system Energy_consumption_model_V3/Simulink Function24 ==
  arr_db : TriggerPort  TriggerType=function-call  IsSimulinkFunction=on  FunctionName=arr_db  FunctionVisibility=scoped  VariantControl=(inherit)
  Digital Clock : DigitalClock  SampleTime=-1
  MATLAB Function : MATLAB Function  TreatAsAtomicUnit=on
  ER : Outport
  wires:
  Digital Clock/1 -> MATLAB Function/1(ct_erdb)
  MATLAB Function/1(ERDB) -> ER/1

== system Energy_consumption_model_V3/Simulink Function25 ==
  msgdb : TriggerPort  TriggerType=function-call  IsSimulinkFunction=on  FunctionName=msgdb  FunctionVisibility=scoped  VariantControl=(inherit)
  Constant : Constant
  Send : Send  OutputPortMessageModes=m
  Out1 : Outport
  wires:
  Constant/1 -> Send/1
  Send/1 -> Out1/1

== system Energy_consumption_model_V3/Simulink Function26 ==
  EC_db : TriggerPort  TriggerType=function-call  IsSimulinkFunction=on  FunctionName=EC_db  FunctionVisibility=scoped  VariantControl=(inherit)
  Digital Clock : DigitalClock  SampleTime=-1
  MATLAB Function : MATLAB Function  TreatAsAtomicUnit=on
  EC : Outport
  wires:
  Digital Clock/1 -> MATLAB Function/1(ct_ecdb)
  MATLAB Function/1(ECDB) -> EC/1

== system Energy_consumption_model_V3/Simulink Function27 ==
  arr_fg : TriggerPort  TriggerType=function-call  IsSimulinkFunction=on  FunctionName=arr_fg  FunctionVisibility=scoped  VariantControl=(inherit)
  Digital Clock : DigitalClock  SampleTime=-1
  MATLAB Function : MATLAB Function  TreatAsAtomicUnit=on
  ER : Outport
  wires:
  Digital Clock/1 -> MATLAB Function/1(ct_erfg)
  MATLAB Function/1(ERFG) -> ER/1

== system Energy_consumption_model_V3/Simulink Function28 ==
  msgfg : TriggerPort  TriggerType=function-call  IsSimulinkFunction=on  FunctionName=msgfg  FunctionVisibility=scoped  VariantControl=(inherit)
  Constant : Constant
  Send : Send  OutputPortMessageModes=m
  Out1 : Outport
  wires:
  Constant/1 -> Send/1
  Send/1 -> Out1/1

== system Energy_consumption_model_V3/Simulink Function29 ==
  EC_fg : TriggerPort  TriggerType=function-call  IsSimulinkFunction=on  FunctionName=EC_fg  FunctionVisibility=scoped  VariantControl=(inherit)
  Digital Clock : DigitalClock  SampleTime=-1
  MATLAB Function : MATLAB Function  TreatAsAtomicUnit=on
  EC : Outport
  wires:
  Digital Clock/1 -> MATLAB Function/1(ct_ecfg)
  MATLAB Function/1(ECFG) -> EC/1

== system Energy_consumption_model_V3/Simulink Function3 ==
  arr_mc2 : TriggerPort  TriggerType=function-call  IsSimulinkFunction=on  FunctionName=arr_mc2  FunctionVisibility=scoped  VariantControl=(inherit)
  Digital Clock : DigitalClock  SampleTime=-1
  MATLAB Function : MATLAB Function  TreatAsAtomicUnit=on
  ER : Outport
  ER1 : Outport  Port=2
  wires:
  Digital Clock/1 -> MATLAB Function/1(ct_ertm2)
  MATLAB Function/1(ERTM2) -> ER1/1, ER/1

== system Energy_consumption_model_V3/Simulink Function30 ==
  arr_wc : TriggerPort  TriggerType=function-call  IsSimulinkFunction=on  FunctionName=arr_wc  FunctionVisibility=scoped  VariantControl=(inherit)
  Digital Clock : DigitalClock  SampleTime=-1
  MATLAB Function : MATLAB Function  TreatAsAtomicUnit=on
  ER : Outport
  wires:
  Digital Clock/1 -> MATLAB Function/1(ct_erwc)
  MATLAB Function/1(ERWC) -> ER/1

== system Energy_consumption_model_V3/Simulink Function31 ==
  msgwc : TriggerPort  TriggerType=function-call  IsSimulinkFunction=on  FunctionName=msgwc  FunctionVisibility=scoped  VariantControl=(inherit)
  Constant : Constant
  Send : Send  OutputPortMessageModes=m
  Out1 : Outport
  wires:
  Constant/1 -> Send/1
  Send/1 -> Out1/1

== system Energy_consumption_model_V3/Simulink Function32 ==
  EC_wc : TriggerPort  TriggerType=function-call  IsSimulinkFunction=on  FunctionName=EC_wc  FunctionVisibility=scoped  VariantControl=(inherit)
  Digital Clock : DigitalClock  SampleTime=-1
  MATLAB Function : MATLAB Function  TreatAsAtomicUnit=on
  EC : Outport
  wires:
  Digital Clock/1 -> MATLAB Function/1(ct_ecwc)
  MATLAB Function/1(ECWC) -> EC/1

== system Energy_consumption_model_V3/Simulink Function33 ==
  arr_l : TriggerPort  TriggerType=function-call  IsSimulinkFunction=on  FunctionName=arr_l  FunctionVisibility=scoped  VariantControl=(inherit)
  Digital Clock : DigitalClock  SampleTime=-1
  MATLAB Function : MATLAB Function  TreatAsAtomicUnit=on
  ER : Outport
  wires:
  Digital Clock/1 -> MATLAB Function/1(ct_erwc)
  MATLAB Function/1(ERWC) -> ER/1

== system Energy_consumption_model_V3/Simulink Function34 ==
  msgl : TriggerPort  TriggerType=function-call  IsSimulinkFunction=on  FunctionName=msgl  FunctionVisibility=scoped  VariantControl=(inherit)
  Constant : Constant
  Send : Send  OutputPortMessageModes=m
  Out1 : Outport
  wires:
  Constant/1 -> Send/1
  Send/1 -> Out1/1

== system Energy_consumption_model_V3/Simulink Function35 ==
  EC_l : TriggerPort  TriggerType=function-call  IsSimulinkFunction=on  FunctionName=EC_l  FunctionVisibility=scoped  VariantControl=(inherit)
  Digital Clock : DigitalClock  SampleTime=-1
  MATLAB Function : MATLAB Function  TreatAsAtomicUnit=on
  EC : Outport
  wires:
  Digital Clock/1 -> MATLAB Function/1(ct_ecwc)
  MATLAB Function/1(ECWC) -> EC/1

== system Energy_consumption_model_V3/Simulink Function4 ==
  msg2 : TriggerPort  TriggerType=function-call  IsSimulinkFunction=on  FunctionName=msg2  FunctionVisibility=scoped  VariantControl=(inherit)
  Constant : Constant
  Send : Send  OutputPortMessageModes=m
  Out1 : Outport
  wires:
  Constant/1 -> Send/1
  Send/1 -> Out1/1

== system Energy_consumption_model_V3/Simulink Function5 ==
  EC_mc2 : TriggerPort  TriggerType=function-call  IsSimulinkFunction=on  FunctionName=EC_mc2  FunctionVisibility=scoped  VariantControl=(inherit)
  Digital Clock : DigitalClock  SampleTime=-1
  MATLAB Function : MATLAB Function  TreatAsAtomicUnit=on
  EC : Outport
  wires:
  Digital Clock/1 -> MATLAB Function/1(ct_ectm2)
  MATLAB Function/1(ECTM2) -> EC/1

== system Energy_consumption_model_V3/Simulink Function6 ==
  arr_mc3 : TriggerPort  TriggerType=function-call  IsSimulinkFunction=on  FunctionName=arr_mc3  FunctionVisibility=scoped  VariantControl=(inherit)
  Digital Clock : DigitalClock  SampleTime=-1
  MATLAB Function : MATLAB Function  TreatAsAtomicUnit=on
  ER : Outport
  ER1 : Outport  Port=2
  wires:
  Digital Clock/1 -> MATLAB Function/1(ct_ertm3)
  MATLAB Function/1(ERTM3) -> ER1/1, ER/1

== system Energy_consumption_model_V3/Simulink Function7 ==
  msg3 : TriggerPort  TriggerType=function-call  IsSimulinkFunction=on  FunctionName=msg3  FunctionVisibility=scoped  VariantControl=(inherit)
  Constant : Constant
  Send : Send  OutputPortMessageModes=m
  Out1 : Outport
  wires:
  Constant/1 -> Send/1
  Send/1 -> Out1/1

== system Energy_consumption_model_V3/Simulink Function8 ==
  EC_mc3 : TriggerPort  TriggerType=function-call  IsSimulinkFunction=on  FunctionName=EC_mc3  FunctionVisibility=scoped  VariantControl=(inherit)
  Digital Clock : DigitalClock  SampleTime=-1
  MATLAB Function : MATLAB Function  TreatAsAtomicUnit=on
  EC : Outport
  wires:
  Digital Clock/1 -> MATLAB Function/1(ct_ectm3)
  MATLAB Function/1(ECTM3) -> EC/1

== system Energy_consumption_model_V3/Simulink Function9 ==
  arr_mc4 : TriggerPort  TriggerType=function-call  IsSimulinkFunction=on  FunctionName=arr_mc4  FunctionVisibility=scoped  VariantControl=(inherit)
  Digital Clock : DigitalClock  SampleTime=-1
  MATLAB Function : MATLAB Function  TreatAsAtomicUnit=on
  ER : Outport
  wires:
  Digital Clock/1 -> MATLAB Function/1(ct_ertm4)
  MATLAB Function/1(ERTM4) -> ER/1

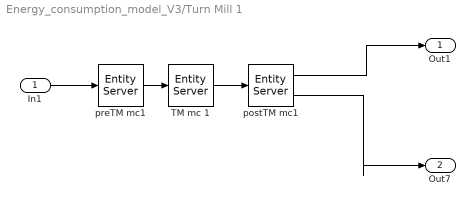
== system Energy_consumption_model_V3/Turn Mill 1 ==
  In1 : Inport
  TM mc 1 : EntityServer  InputPortMessageModes=m  OutputPortMessageModes=m  Capacity=1  ServiceTimeSource=MATLAB action  ServiceTimeAction=|  EntryAction=EC_mc1()  ServiceCompleteAction=EC_mc1()
      | coder.extrinsic("makedist")
      | pd = double(10);
      |  %rng('shuffle');
      | pd=random(makedist('Triangular','a',0.75,'b',5.56,'c',6.75),[1,1]);
      | dt = pd;
  postTM mc1 : EntityServer  InputPortMessageModes=m  OutputPortMessageModes=n,m  Capacity=1  ServiceTimeSource=MATLAB action  ServiceTimeAction=dt = 0.25;  ServiceCompleteAction=arr_mc1()  ExitAction=msg1()  NumberEntitiesDeparted=on
      settings: OutputPortMap=o0,o9
  preTM mc1 : EntityServer  InputPortMessageModes=m  OutputPortMessageModes=m  Capacity=1  ServiceTimeSource=MATLAB action  ServiceTimeAction=dt = 0.25;  EntryAction=|
      | arr_mc1()
      | %Time = 1250
  Out1 : Outport
  Out7 : Outport  Port=2
  wires:
  preTM mc1/1 -> TM mc 1/1
  TM mc 1/1 -> postTM mc1/1
  In1/1 -> preTM mc1/1
  postTM mc1/2 -> Out7/1
  postTM mc1/1 -> Out1/1

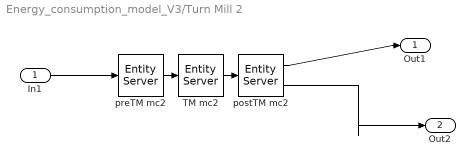
== system Energy_consumption_model_V3/Turn Mill 2 ==
  In1 : Inport
  TM mc2 : EntityServer  InputPortMessageModes=m  OutputPortMessageModes=m  Capacity=1  ServiceTimeSource=MATLAB action  ServiceTimeAction=|  EntryAction=EC_mc2()  ServiceCompleteAction=EC_mc2()
      | coder.extrinsic("makedist")
      | pd = double(10);
      |  %rng('shuffle');
      | pd=random(makedist('Triangular','a',0.75,'b',5.33,'c',7.75),[1,1]);
      | dt = pd;
  postTM mc2 : EntityServer  InputPortMessageModes=m  OutputPortMessageModes=n,m  Capacity=1  ServiceTimeSource=MATLAB action  ServiceTimeAction=dt = 0.25;  ServiceCompleteAction=arr_mc2()  ExitAction=msg2()  NumberEntitiesDeparted=on
      settings: OutputPortMap=o0,o9
  preTM mc2 : EntityServer  InputPortMessageModes=m  OutputPortMessageModes=m  Capacity=1  ServiceTimeSource=MATLAB action  ServiceTimeAction=dt = 0.25;  EntryAction=arr_mc2()
  Out1 : Outport
  Out2 : Outport  Port=2
  wires:
  postTM mc2/1 -> Out1/1
  TM mc2/1 -> postTM mc2/1
  preTM mc2/1 -> TM mc2/1
  In1/1 -> preTM mc2/1
  postTM mc2/2 -> Out2/1

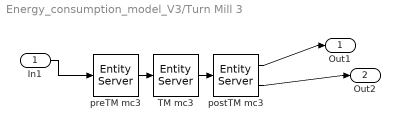
== system Energy_consumption_model_V3/Turn Mill 3 ==
  In1 : Inport
  TM mc3 : EntityServer  InputPortMessageModes=m  OutputPortMessageModes=m  Capacity=1  ServiceTimeSource=MATLAB action  ServiceTimeAction=|  EntryAction=EC_mc3()  ServiceCompleteAction=EC_mc3()
      | coder.extrinsic("makedist")
      | pd = double(10);
      |  %rng('shuffle');
      | pd=random(makedist('Triangular','a',0.75,'b',5.06,'c',8.75),[1,1]);
      | dt = pd;
  postTM mc3 : EntityServer  InputPortMessageModes=m  OutputPortMessageModes=n,m  Capacity=1  ServiceTimeSource=MATLAB action  ServiceTimeAction=dt = 0.25;  ServiceCompleteAction=arr_mc3()  ExitAction=msg3()  NumberEntitiesDeparted=on
      settings: OutputPortMap=o0,o9
  preTM mc3 : EntityServer  InputPortMessageModes=m  OutputPortMessageModes=m  Capacity=1  ServiceTimeSource=MATLAB action  ServiceTimeAction=dt = 0.25;  EntryAction=arr_mc3()
  Out1 : Outport
  Out2 : Outport  Port=2
  wires:
  postTM mc3/2 -> Out2/1
  TM mc3/1 -> postTM mc3/1
  preTM mc3/1 -> TM mc3/1
  postTM mc3/1 -> Out1/1
  In1/1 -> preTM mc3/1

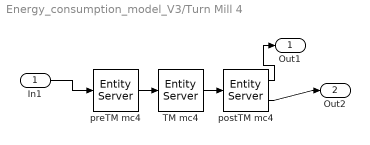
== system Energy_consumption_model_V3/Turn Mill 4 ==
  In1 : Inport
  TM mc4 : EntityServer  InputPortMessageModes=m  OutputPortMessageModes=m  Capacity=1  ServiceTimeSource=MATLAB action  ServiceTimeAction=|  EntryAction=EC_mc4()  ServiceCompleteAction=EC_mc4()
      | coder.extrinsic("makedist")
      | pd = double(10)
      | % rng('shuffle');
      | pd=random(makedist('Triangular','a',0.8,'b',3.63,'c',8),[1,1])
      | dt = pd
  postTM mc4 : EntityServer  InputPortMessageModes=m  OutputPortMessageModes=n,m  Capacity=1  ServiceTimeSource=MATLAB action  ServiceTimeAction=dt = 0.25;  ServiceCompleteAction=arr_mc4()  ExitAction=msg4()  NumberEntitiesDeparted=on
      settings: OutputPortMap=o0,o9
  preTM mc4 : EntityServer  InputPortMessageModes=m  OutputPortMessageModes=m  Capacity=1  ServiceTimeSource=MATLAB action  ServiceTimeAction=dt = 0.25;  EntryAction=arr_mc4()
  Out1 : Outport
  Out2 : Outport  Port=2
  wires:
  preTM mc4/1 -> TM mc4/1
  TM mc4/1 -> postTM mc4/1
  postTM mc4/1 -> Out1/1
  In1/1 -> preTM mc4/1
  postTM mc4/2 -> Out2/1

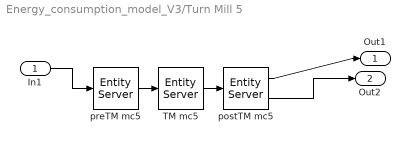
== system Energy_consumption_model_V3/Turn Mill 5 ==
  In1 : Inport
  TM mc5 : EntityServer  InputPortMessageModes=m  OutputPortMessageModes=m  Capacity=1  ServiceTimeSource=MATLAB action  ServiceTimeAction=|  EntryAction=EC_mc5()  ServiceCompleteAction=EC_mc5()
      | coder.extrinsic("makedist")
      | pd = double(10)
      | % rng('shuffle');
      | pd=random(makedist('Triangular','a',0.66,'b',4.66,'c',8.25),[1,1])
      | dt = pd
  postTM mc5 : EntityServer  InputPortMessageModes=m  OutputPortMessageModes=n,m  Capacity=1  ServiceTimeSource=MATLAB action  ServiceTimeAction=dt = 0.25;  ServiceCompleteAction=arr_mc5()  ExitAction=msg5()  NumberEntitiesDeparted=on
      settings: OutputPortMap=o0,o9
  preTM mc5 : EntityServer  InputPortMessageModes=m  OutputPortMessageModes=m  Capacity=1  ServiceTimeSource=MATLAB action  ServiceTimeAction=dt = 0.25;  EntryAction=arr_mc5()
  Out1 : Outport
  Out2 : Outport  Port=2
  wires:
  TM mc5/1 -> postTM mc5/1
  postTM mc5/1 -> Out1/1
  preTM mc5/1 -> TM mc5/1
  In1/1 -> preTM mc5/1
  postTM mc5/2 -> Out2/1

== system Energy_consumption_model_V3/Wire Cutting ==
  In1 : Inport
  Wire cut : EntityServer  InputPortMessageModes=m  OutputPortMessageModes=m  Capacity=1  ServiceTimeSource=MATLAB action  ServiceTimeAction=|  EntryAction=|  ServiceCompleteAction=EC_wc()
      ServiceTimeAction=|
      | coder.extrinsic("makedist")
      | pd = double(10)
      | pd=random(makedist('Triangular','a',0.75,'b',5.63,'c',7.75),[1,1])
      | dt = pd
      EntryAction=|
      | entity.Route = 3
      | EC_wc()
  postWC : EntityServer  InputPortMessageModes=m  OutputPortMessageModes=n,m  Capacity=1  ServiceTimeSource=MATLAB action  ServiceTimeAction=dt = 0.25;  ServiceCompleteAction=arr_wc()  ExitAction=msgwc()  NumberEntitiesDeparted=on
      settings: OutputPortMap=o0,o9
  preWC : EntityServer  InputPortMessageModes=m  OutputPortMessageModes=m  Capacity=1  ServiceTimeSource=MATLAB action  ServiceTimeAction=dt = 0.25;  EntryAction=arr_wc()
  Out1 : Outport
  Out2 : Outport  Port=2
  wires:
  preWC/1 -> Wire cut/1
  Wire cut/1 -> postWC/1
  postWC/1 -> Out2/1
  In1/1 -> preWC/1
  postWC/2 -> Out1/1
